simulink model "Magnetic_Torquers_detumbling"  (R2015b)
settings: Solver=VariableStepAuto  StartTime=0.0  StopTime=stop_time  RelTol=1e-6
values from neighbouring files (symbols this model uses):
  alpha_0 = 5.1191    [Main_magnetic_torquers_detumbling.m]
  B_quaternion = [zeros(4,3);diag([1/I_x 1/I_y 1/I_z])]    [Main_magnetic_torquers_detumbling.m]
  i = 87*180/pi    (= 4984.73281764)    [Main_magnetic_torquers_detumbling.m]
  I_x = 1    [Main_magnetic_torquers_detumbling.m]
  I_y = 0.5    [Main_magnetic_torquers_detumbling.m]
  I_z = 0.7    [Main_magnetic_torquers_detumbling.m]
  k = 1    [Main_magnetic_torquers_detumbling.m]
  m_E = 7.77e15    (= 7.77e+15)    [Main_magnetic_torquers_detumbling.m]
  n = sqrt(G*M_E/R^3)    [Main_magnetic_torquers_detumbling.m]
  Omega = 0    [Main_magnetic_torquers_detumbling.m]
  omega_e = 360.99/180*pi/(24*60*60)    (= 7.29220378099e-05)    [Main_magnetic_torquers_detumbling.m]
  phi = 5.6913    [Main_magnetic_torquers_detumbling.m]
  R = R_E+h    (= 6821000)    [Main_magnetic_torquers_detumbling.m]
  theta_m = 169.7/180*pi    (= 2.96182374063)    [Main_magnetic_torquers_detumbling.m]
  X_0 = [epsilon_0 ... (first row only)    [Main_magnetic_torquers_detumbling.m]
libraries: vrlib x2
settings Model: Creator=Krunal's PC  LastModifiedBy=Krunal's PC

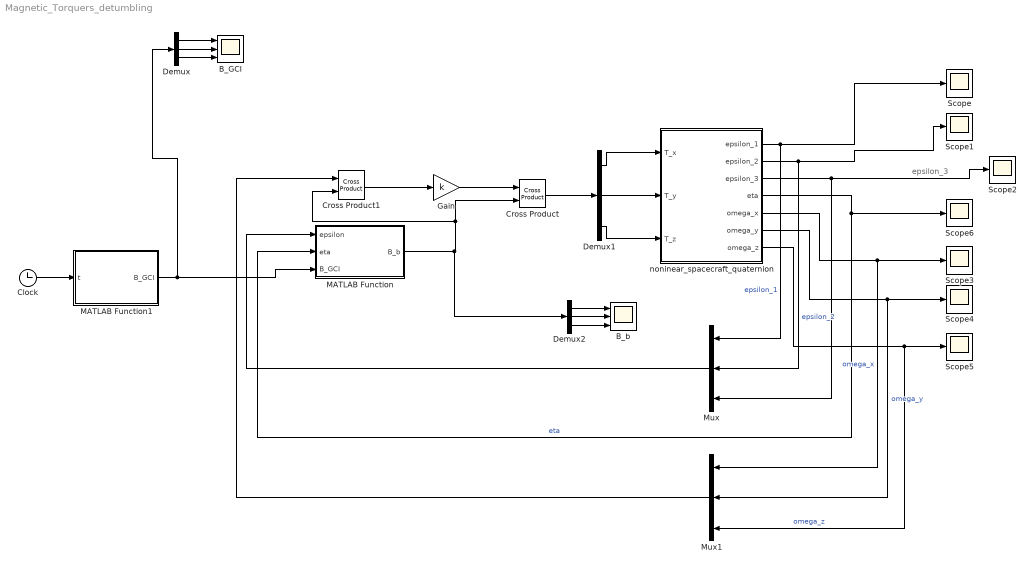
== system Magnetic_Torquers_detumbling ==
  note: epsilon_3
  B_GCI : Scope  NumInputPorts=3
  B_b : Scope  NumInputPorts=3
  Clock : Clock
  Cross Product : vrlib/Utilities/Cross Product
  Cross Product1 : vrlib/Utilities/Cross Product
  Demux : Demux  Outputs=3
  Demux1 : Demux  Outputs=3
  Demux2 : Demux  Outputs=3
  Gain : Gain  Gain=k
  MATLAB Function : MATLAB Function  TreatAsAtomicUnit=on
  MATLAB Function1 : MATLAB Function  TreatAsAtomicUnit=on
  Mux : Mux  Inputs=3
  Mux1 : Mux  Inputs=3
  Scope{,1..6} (7 alike) : Scope
  noninear_spacecraft_quaternion : Subsystem
  wires:
  noninear_spacecraft_quaternion/1(epsilon_1) -> Mux/1, Scope/1  "epsilon_1"
  noninear_spacecraft_quaternion/2(epsilon_2) -> Mux/2, Scope1/1  "epsilon_2"
  noninear_spacecraft_quaternion/3(epsilon_3) -> Mux/3, Scope2/1
  noninear_spacecraft_quaternion/7(omega_z) -> Mux1/3, Scope5/1  "omega_z"
  noninear_spacecraft_quaternion/6(omega_y) -> Mux1/2, Scope4/1  "omega_y"
  noninear_spacecraft_quaternion/5(omega_x) -> Mux1/1, Scope3/1  "omega_x"
  noninear_spacecraft_quaternion/4(eta) -> MATLAB Function/2(eta), Scope6/1  "eta"
  Demux1/1 -> noninear_spacecraft_quaternion/1(T_x)
  Demux1/2 -> noninear_spacecraft_quaternion/2(T_y)
  Demux1/3 -> noninear_spacecraft_quaternion/3(T_z)
  Cross Product/1 -> Demux1/1
  MATLAB Function/1(B_b) -> Demux2/1, Cross Product1/2, Cross Product/2
  Mux/1 -> MATLAB Function/1(epsilon)
  MATLAB Function1/1(B_GCI) -> Demux/1, MATLAB Function/3(B_GCI)
  Clock/1 -> MATLAB Function1/1(t)
  Demux/1 -> B_GCI/1
  Demux/2 -> B_GCI/2
  Demux/3 -> B_GCI/3
  Demux2/1 -> B_b/1
  Demux2/2 -> B_b/2
  Demux2/3 -> B_b/3
  Gain/1 -> Cross Product/1
  Cross Product1/1 -> Gain/1
  Mux1/1 -> Cross Product1/1

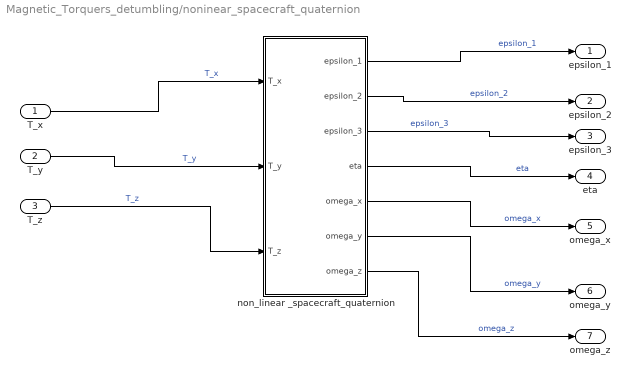
== system Magnetic_Torquers_detumbling/noninear_spacecraft_quaternion ==
  T_x : Inport
  T_y : Inport  Port=2
  T_z : Inport  Port=3
  non_linear _spacecraft_quaternion : Subsystem
  epsilon_1 : Outport
  epsilon_2 : Outport  Port=2
  epsilon_3 : Outport  Port=3
  eta : Outport  Port=4
  omega_x : Outport  Port=5
  omega_y : Outport  Port=6
  omega_z : Outport  Port=7
  wires:
  T_x/1 -> non_linear _spacecraft_quaternion/1(T_x)  "T_x"
  T_y/1 -> non_linear _spacecraft_quaternion/2(T_y)  "T_y"
  T_z/1 -> non_linear _spacecraft_quaternion/3(T_z)  "T_z"
  non_linear _spacecraft_quaternion/1(epsilon_1) -> epsilon_1/1  "epsilon_1"
  non_linear _spacecraft_quaternion/2(epsilon_2) -> epsilon_2/1  "epsilon_2"
  non_linear _spacecraft_quaternion/3(epsilon_3) -> epsilon_3/1  "epsilon_3"
  non_linear _spacecraft_quaternion/4(eta) -> eta/1  "eta"
  non_linear _spacecraft_quaternion/5(omega_x) -> omega_x/1  "omega_x"
  non_linear _spacecraft_quaternion/6(omega_y) -> omega_y/1  "omega_y"
  non_linear _spacecraft_quaternion/7(omega_z) -> omega_z/1  "omega_z"

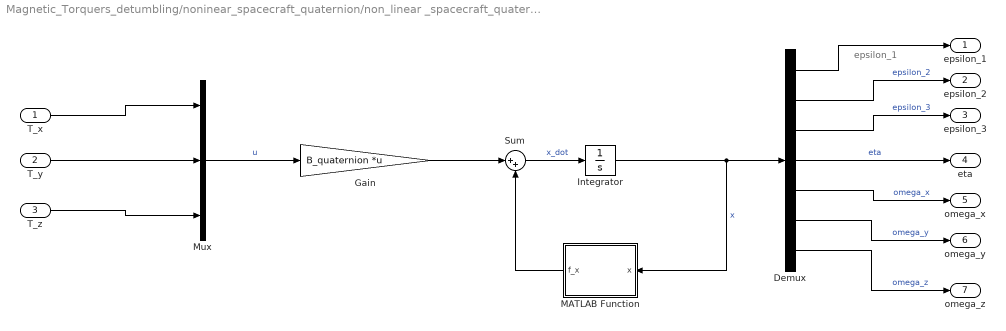
== system Magnetic_Torquers_detumbling/noninear_spacecraft_quaternion/non_linear _spacecraft_quaternion ==
  note: epsilon_1
  T_x : Inport
  T_y : Inport  Port=2
  T_z : Inport  Port=3
  Demux : Demux  Outputs=7
  Gain : Gain  Gain=B_quaternion  Multiplication=Matrix(K*u)
  Integrator : Integrator  InitialCondition=X_0  ZeroCross=off
  MATLAB Function : MATLAB Function  TreatAsAtomicUnit=on
  Mux : Mux  Inputs=3
  Sum : Sum  Inputs=|++
  epsilon_1 : Outport
  epsilon_2 : Outport  Port=2
  epsilon_3 : Outport  Port=3
  eta : Outport  Port=4
  omega_x : Outport  Port=5
  omega_y : Outport  Port=6
  omega_z : Outport  Port=7
  wires:
  T_y/1 -> Mux/2
  Mux/1 -> Gain/1  "u"
  Demux/2 -> epsilon_2/1  "epsilon_2"
  Demux/3 -> epsilon_3/1  "epsilon_3"
  T_x/1 -> Mux/1
  T_z/1 -> Mux/3
  Demux/1 -> epsilon_1/1
  Gain/1 -> Sum/1
  Sum/1 -> Integrator/1  "x_dot"
  Integrator/1 -> MATLAB Function/1(x), Demux/1  "x"
  MATLAB Function/1(f_x) -> Sum/2
  Demux/4 -> eta/1  "eta"
  Demux/5 -> omega_x/1  "omega_x"
  Demux/6 -> omega_y/1  "omega_y"
  Demux/7 -> omega_z/1  "omega_z"

== matlab function Magnetic_Torquers_detumbling/MATLAB Function ==
  data: epsilon input; B_b output; eta input; B_GCI input
function B_b = B_b(epsilon,eta,B_GCI)

epsilon_cross=[0 epsilon(3,1) epsilon(2,1);
              epsilon(3,1) 0 -epsilon(1,1);
              -epsilon(2,1) epsilon(1,1) 0;]
C=(2*eta^2-1)*eye(3)+2*epsilon*(epsilon')-2*eta*epsilon_cross

B_b = C*B_GCI;

== matlab function Magnetic_Torquers_detumbling/noninear_spacecraft_quaternion/non_linear _spacecraft_quaternion/MATLAB Function ==
  data: x input; f_x output; I_x parameter; I_y parameter; I_z parameter
function f_x = fcn(x,I_x,I_y,I_z)

epsilon=zeros(3,1); %initialization
epsilon(1,1)=x(1);
epsilon(2,1)=x(2);
epsilon(3,1)=x(3);
eta=x(4);
omega_x=x(5);
omega_y=x(6);
omega_z=x(7);

epsilon_cross= [0 -epsilon(3,1) epsilon(2,1);
                epsilon(3,1) 0 -epsilon(1,1);
                -epsilon(2,1) epsilon(1,1) 0]
omega=[omega_x;
       omega_y;
       omega_z];
            
epsilon_dot= 1/2*(eta*eye(3)+epsilon_cross)*omega

eta_dot=1/2*epsilon'*omega;

f_x=zeros(7,1);

f_x(1,1)= epsilon_dot(1,1);
f_x(2,1)= epsilon_dot(2,1);
f_x(3,1)= epsilon_dot(3,1);
f_x(4,1)= eta_dot;
f_x(5,1)= (I_y-I_z)/I_x*omega_y*omega_z;
f_x(6,1)= (I_z-I_x)/I_y*omega_x*omega_z;
f_x(7,1)= (I_x-I_y)/I_z*omega_x*omega_y;

== matlab function Magnetic_Torquers_detumbling/MATLAB Function1 ==
  data: t input; B_GCI output; m_E parameter; theta_m parameter; omega_e parameter; R parameter; alpha_0 parameter; n parameter; phi parameter; i parameter; Omega parameter
function B_GCI= B_GCI(t,m_E,theta_m,omega_e,R,alpha_0,n,phi,i,Omega)

m_E_GCI=m_E*[sin(theta_m)*cos(omega_e*t+alpha_0);
             sin(theta_m)*sin(omega_e*t+alpha_0);
             cos(theta_m)];
r_o=[R*cos(n*t+phi);
     R*sin(n*t+phi);
     0];
R_x_minus_i= [1 0 0;
              0 cos(i) -sin(i);
              0 sin(i) cos(i)];
R_z_minus_Omega= [cos(Omega) -sin(Omega) 0;
                  sin(Omega) cos(Omega) 0;
                  0 0 1];
r_GCI= R_z_minus_Omega*R_x_minus_i*r_o;

B_GCI=(3*(m_E_GCI'*r_GCI)*r_GCI-R^2*m_E_GCI)/R^5 ;
